simulink model "XplaneControlInterface"  (R2024b)
settings: Solver=FixedStepAuto  StartTime=0.0  StopTime=inf  FixedStep=0.02  RelTol=1e-3
libraries: dspnetwork x3, instrumentseriallib x2, etargetslib x2, sldrtlib x2, svdutilitieslib x1, slpidlib x1
settings Model: PacingRate=10  Creator=정예린  LastModifiedBy=banana99ou
settings RTWCC: GPUComputeCapability=3.5

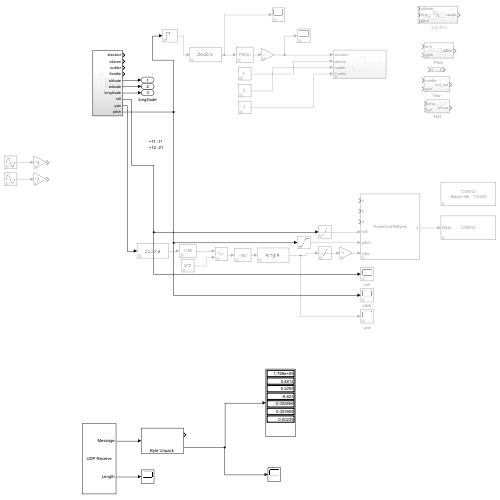
[thumbnail: Simulink's stored preview of the top-level diagram]
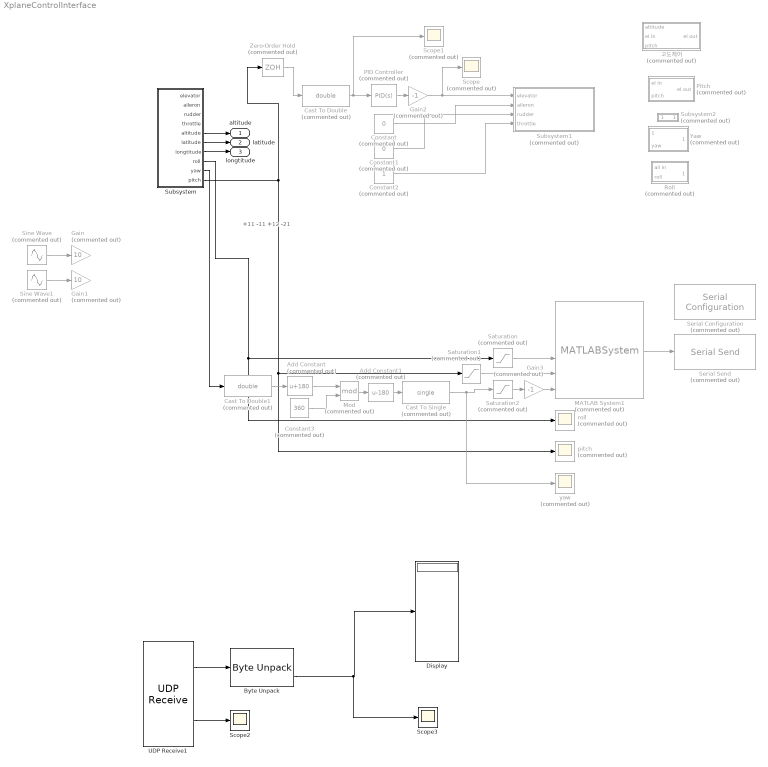
== system XplaneControlInterface ==
  note: +11 -11
      | +12 -21
  Add Constant : Bias  Commented=on  Bias=180  SaturateOnIntegerOverflow=off
  Add Constant1 : Bias  Commented=on  Bias=-180  SaturateOnIntegerOverflow=off
  Byte Unpack : svdutilitieslib/Byte Unpack  dimensions={[1],[7]}  datatypes={'single','single'}  byteAlign=4  blockPlatform=arduinoert
  Cast To Double : DataTypeConversion  Commented=on  OutDataTypeStr=double  SaturateOnIntegerOverflow=off  RndMeth=Floor
  Cast To Double1 : DataTypeConversion  Commented=on  OutDataTypeStr=double  SaturateOnIntegerOverflow=off  RndMeth=Floor
  Cast To Single : DataTypeConversion  Commented=on  OutDataTypeStr=single  SaturateOnIntegerOverflow=off  RndMeth=Floor
  Constant : Constant  Commented=on  Value=0
  Constant1 : Constant  Commented=on  Value=0
  Constant2 : Constant  Commented=on
  Constant3 : Constant  Commented=on  Value=360
  Display : Display
  Gain : Gain  Commented=on  Gain=10
  Gain1 : Gain  Commented=on  Gain=10
  Gain2 : Gain  Commented=on  Gain=-1
  Gain3 : Gain  Commented=on  Gain=-1
  MATLAB System1 : MATLABSystem  Commented=on  System=PoseCmdToBytes  Precision=3  MaxLen=128  PadByte=10  SimulateUsing=Code generation
      mask Type: PoseCmdToBytes
      mask Display:
      | disp('PoseCmdToBytes');
      | port_label('input',1,'x');
      | port_label('input',2,'y');
      | port_label('input',3,'z');
      | port_label('input',4,'roll');
      | port_label('input',5,'pitch');
      | port_label('input',6,'yaw');
      | port_label('output',1,'y');
  Mod : Math  Commented=on  Operator=mod
  PID Controller : slpidlib/PID Controller  Commented=on  Controller=PID  Form=Parallel  TimeDomain=Continuous-time  UseExternalTs=off  SampleTime=-1  IntegratorMethod=Forward Euler  FilterMethod=Forward Euler  ControllerParametersSource=internal  P=4  I=0  UseKiTs=off  D=0  UseExternalDerivativeSource=off  N=100  UseFilter=on  TunerSelectOption=Transfer Function Based (PID Tuner App)  InitialConditionSource=internal  InitialConditionForIntegrator=0  InitialConditionForFilter=0  DifferentiatorICPrevScaledInput=0  ExternalReset=none  TrackingMode=off  Kt=1  LimitOutput=off  SatLimitsSource=internal  UpperSaturationLimit=inf  LowerSaturationLimit=-inf  LinearizeAsGain=on  AntiWindupMode=none  Kb=1  LimitIntegrator=off  UpperIntegratorSaturationLimit=inf  LowerIntegratorSaturationLimit=-inf  POutMin=[]  POutMax=[]  IOutMin=[]  IOutMax=[]  DOutMin=[]  DOutMax=[]  NOutMin=[]  NOutMax=[]  SumOutMin=[]  SumOutMax=[]  SaturationOutMin=[]  SaturationOutMax=[]  PParamMin=[]  PParamMax=[]  IParamMin=[]  IParamMax=[]  DParamMin=[]  DParamMax=[]  NParamMin=[]  NParamMax=[]  KbParamMin=[]  KbParamMax=[]  KtParamMin=[]  KtParamMax=[]  KbOutMin=[]  KbOutMax=[]  KtOutMin=[]  KtOutMax=[]  IntegratorOutMin=[]  IntegratorOutMax=[]  FilterOutMin=[]  FilterOutMax=[]  SumI1OutMin=[]  SumI1OutMax=[]  SumI2OutMin=[]  SumI2OutMax=[]  SumI3OutMin=[]  SumI3OutMax=[]  SumI4OutMin=[]  SumI4OutMax=[]  SumDOutMin=[]  SumDOutMax=[]  DifferentiatorOutMin=[]  DifferentiatorOutMax=[]  FilterDiffOutCoefMin=[]  FilterDiffOutCoefMax=[]  ReciprocalOutMin=[]  ReciprocalOutMax=[]  SumDenOutMin=[]  SumDenOutMax=[]  SumNumOutMin=[]  SumNumOutMax=[]  DivideOutMin=[]  DivideOutMax=[]  UdiffTsProdOutMin=[]  UdiffTsProdOutMax=[]  NTsProdOutMin=[]  NTsProdOutMax=[]  UintegralTsProdOutMin=[]  UintegralTsProdOutMax=[]  UngainTsProdOutMin=[]  UngainTsProdOutMax=[]  ClampingZeroOutDataTypeStr=Inherit: Inherit via back propagation  ClampingZeroOutMin=[]  ClampingZeroOutMax=[]  FilterDenConstantOutDataTypeStr=Inherit: Inherit via back propagation  FilterDenConstantOutMin=[]  FilterDenConstantOutMax=[]  PCopyOutDataTypeStr=Inherit: Inherit via back propagation  PCopyOutMin=[]  PCopyOutMax=[]  NCopyOutDataTypeStr=Inherit: Inherit via back propagation  NCopyOutMin=[]  NCopyOutMax=[]  IntegratorContinuousStateAttributes=''  IntegratorStateMustResolveToSignalObject=off  IntegratorRTWStateStorageClass=Auto  FilterContinuousStateAttributes=''  FilterStateMustResolveToSignalObject=off  FilterRTWStateStorageClass=Auto  ParallelPVariant=InternalParameters  IdealPVariant=Disabled  IVariant=InternalParameters  DVariant=InternalParameters  IntegratorVariant=Continuous  SatVariant=Disabled  AWVariant=Passthrough  PCopyVariant=Disabled  TRVariant=Disabled  FdbkBlocksVariant=Forward  IdealPFdbkVariant=Disabled  SatFdbkVariant=Disabled  DerivativeFilterVariant=ContFilter  NVariant=InternalParameters  NCopyVariant=Disabled  FilterICVariant=InternalICsFilter  IntegratorICVariant=InternalICs  ExternalResetVariant=Disabled  TRSumVariant=Passthrough  SumFdbkVariant=Disabled  SumVariant=Sum_PID  TsampFilterVariant=InternalTs  TsampNgainVariant=Passthrough  TsampIntegralVariant=Disabled_SignalSpec  ExternalSaturationOutDataTypeStr=Inherit: Same as second input  DerivativeSourceVariant=ErrorSignal  PreIntVariant=InternalPreInt
  Pitch : Subsystem  Commented=on
  Roll : Subsystem  Commented=on
  Saturation : Saturate  Commented=on  UpperLimit=11  LowerLimit=-11
  Saturation1 : Saturate  Commented=on  UpperLimit=12  LowerLimit=-21
  Saturation2 : Saturate  Commented=on  UpperLimit=20  LowerLimit=-20
  Scope : Scope  Commented=on
  Scope1 : Scope  Commented=on
  Scope2 : Scope
  Scope3 : Scope
  Serial Configuration : instrumentseriallib/Serial Configuration  Priority=-200000  Commented=on  PortSel=COM12  Port=COM12  ComPort=COM12  BaudRate=115200  DataBits=8  Parity=none  StopBits=1  ByteOrder=little-endian  FlowControl=none  Timeout=10  SimulateUsing=Interpreted execution  BlockInModel=on  aMode=1
  Serial Send : instrumentseriallib/Serial Send  Priority=1  Commented=on  PortSel=COM12  Port=COM12  ComPort=COM12  Header=[]  Terminator=<none>  CustomTerminator=[]  EnableBlockingMode=on  SimulateUsing=Interpreted execution  BlockInModel=on  aMode=1
  Sine Wave : Sin  Commented=on  Frequency=0.25  SampleTime=0
  Sine Wave1 : Sin  Commented=on  Frequency=0.25  Phase=1.5708  SampleTime=0
  Subsystem : Subsystem
  Subsystem1 : Subsystem  Commented=on
  Subsystem2 : Subsystem  Commented=on
  UDP Receive1 : dspnetwork/UDP Receive  localURL='0.0.0.0'  localPort=32901  remoteURL='0.0.0.0'  remotePort=-1  recvBufferSize=8192  dims=32  signalDatatype=uint8  isComplex=off  isVarSize=off  showBlockingTime=off  blockingTime=0  sampletime=inf  blockPlatform=[]
  Yaw : Subsystem  Commented=on
  Zero-Order Hold : ZeroOrderHold  Commented=on  SampleTime=-1
  pitch : Scope  Commented=on
  roll : Scope  Commented=on
  yaw : Scope  Commented=on
  고도제어 : Subsystem  Commented=on
  altitude : Outport
  latitude : Outport  Port=2
  longtitude : Outport  Port=3
  wires:
  MATLAB System1/1 -> Serial Send/1
  Sine Wave/1 -> Gain/1
  Sine Wave1/1 -> Gain1/1
  Subsystem/8(roll) -> roll/1, Saturation/1
  Subsystem/10(pitch) -> Zero-Order Hold/1, pitch/1, Saturation1/1
  Subsystem/7(longtitude) -> longtitude/1
  Subsystem/6(latitude) -> latitude/1
  Subsystem/5(altitude) -> altitude/1
  Constant/1 -> Subsystem1/2(aileron)
  Constant1/1 -> Subsystem1/3(rudder)
  Constant2/1 -> Subsystem1/4(throttle)
  PID Controller/1 -> Gain2/1
  Cast To Double/1 -> Scope1/1, PID Controller/1
  Zero-Order Hold/1 -> Cast To Double/1
  Gain2/1 -> Scope/1, Subsystem1/1(elevator)
  Saturation/1 -> MATLAB System1/4
  Saturation2/1 -> Gain3/1
  Saturation1/1 -> MATLAB System1/5
  Subsystem/9(yaw) -> Cast To Double1/1
  Mod/1 -> Add Constant1/1
  Add Constant/1 -> Mod/1
  Constant3/1 -> Mod/2
  Cast To Double1/1 -> Add Constant/1
  Cast To Single/1 -> yaw/1, Saturation2/1
  Add Constant1/1 -> Cast To Single/1
  Gain3/1 -> MATLAB System1/6
  UDP Receive1/1 -> Byte Unpack/1
  UDP Receive1/2 -> Scope2/1
  Byte Unpack/2 -> Scope3/1, Display/1

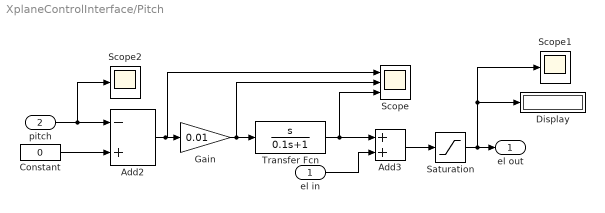
== system XplaneControlInterface/Pitch ==
  el in : Inport
  pitch : Inport  Port=2
  Add2 : Sum  Inputs=-+
  Add3 : Sum
  Constant : Constant  Value=0
  Display : Display
  Gain : Gain  Gain=0.01
  Saturation : Saturate  UpperLimit=1  LowerLimit=-1
  Scope : Scope  NumInputPorts=3
  Scope1 : Scope
  Scope2 : Scope
  Transfer Fcn : TransferFcn  Numerator=[1 0]  Denominator=[0.1 1]
  el out : Outport
  wires:
  el in/1 -> Add3/2
  Add3/1 -> Saturation/1
  Saturation/1 -> Scope1/1, Display/1, el out/1
  Gain/1 -> Scope/2, Transfer Fcn/1
  Add2/1 -> Scope/1, Gain/1
  Transfer Fcn/1 -> Scope/3, Add3/1
  Constant/1 -> Add2/2
  pitch/1 -> Scope2/1, Add2/1

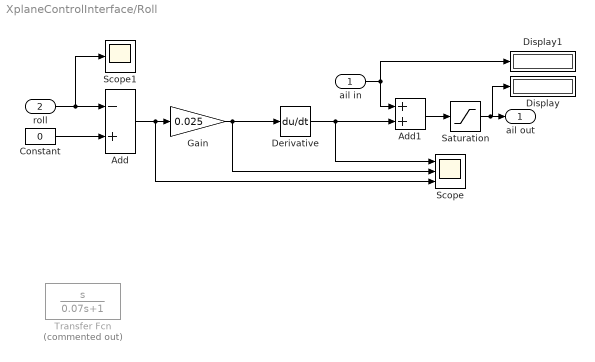
== system XplaneControlInterface/Roll ==
  ail in : Inport
  roll : Inport  Port=2
  Add : Sum  Inputs=-+
  Add1 : Sum
  Constant : Constant  Value=0
  Derivative : Derivative  CoefficientInTFapproximation=0.07
  Display : Display
  Display1 : Display
  Gain : Gain  Gain=0.025
  Saturation : Saturate  UpperLimit=1  LowerLimit=-1
  Scope : Scope  NumInputPorts=3
  Scope1 : Scope
  Transfer Fcn : TransferFcn  Commented=on  Numerator=[1 0]  Denominator=[0.07 1]
  ail out : Outport
  wires:
  Constant/1 -> Add/2
  Add/1 -> Scope/3, Gain/1
  Add1/1 -> Saturation/1
  ail in/1 -> Add1/1, Display1/1
  Saturation/1 -> ail out/1, Display/1
  roll/1 -> Scope1/1, Add/1
  Gain/1 -> Derivative/1, Scope/2
  Derivative/1 -> Scope/1, Add1/2

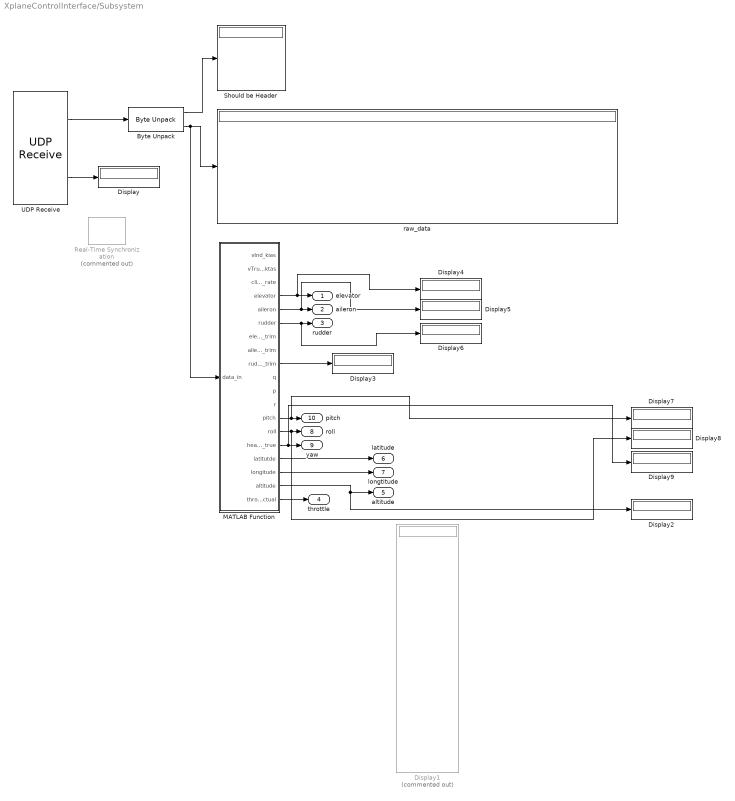
== system XplaneControlInterface/Subsystem ==
  Byte Unpack : etargetslib/Byte Unpack  dimensions={5,[9,8]}  datatypes={'uint8','single'}  byteAlign=1
  Display{,2..9} (9 alike) : Display
  Display1 : Display  Commented=on
  MATLAB Function : MATLAB Function  TreatAsAtomicUnit=on
  Real-Time Synchronization : sldrtlib/Real-Time Synchronization  Commented=on  SampleTime=0.1  MaxMissedTicks=10  ShowMissedTicks=off  YieldWhenWaiting=off
  Should be Header : Display
  UDP Receive : dspnetwork/UDP Receive  localURL='0.0.0.0'  localPort=49004  remoteURL='127.0.0.1'  remotePort=-1  recvBufferSize=8192  dims=293  signalDatatype=uint8  isComplex=off  isVarSize=off  showBlockingTime=off  blockingTime=0  sampletime=inf  blockPlatform=[]
  raw_data : Display
  elevator : Outport
  aileron : Outport  Port=2
  rudder : Outport  Port=3
  throttle : Outport  Port=4
  altitude : Outport  Port=5
  latitude : Outport  Port=6
  longtitude : Outport  Port=7
  roll : Outport  Port=8
  yaw : Outport  Port=9
  pitch : Outport  Port=10
  wires:
  Byte Unpack/1 -> Should be Header/1
  Byte Unpack/2 -> MATLAB Function/1(data_in), raw_data/1
  UDP Receive/2 -> Display/1
  UDP Receive/1 -> Byte Unpack/1
  MATLAB Function/4(elevator) -> Display4/1, elevator/1
  MATLAB Function/5(aileron) -> Display5/1, aileron/1
  MATLAB Function/6(rudder) -> Display6/1, rudder/1
  MATLAB Function/18(altitude) -> altitude/1, Display2/1
  MATLAB Function/19(throttle_actual) -> throttle/1
  MATLAB Function/16(latitutde) -> latitude/1
  MATLAB Function/17(longitude) -> longtitude/1
  MATLAB Function/14(roll) -> Display8/1, roll/1
  MATLAB Function/15(heading_true) -> Display9/1, yaw/1
  MATLAB Function/9(rudder_trim) -> Display3/1
  MATLAB Function/13(pitch) -> Display7/1, pitch/1

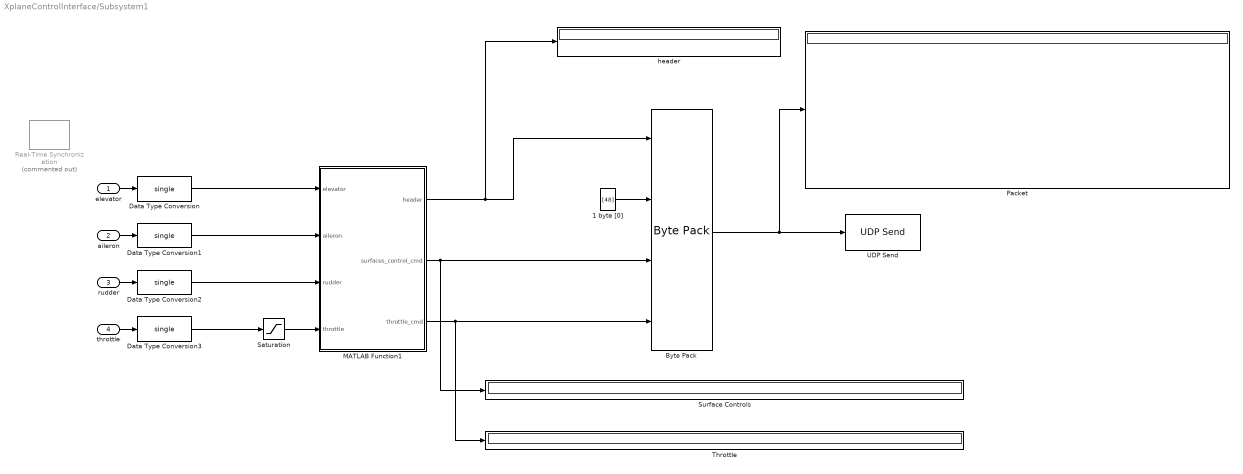
== system XplaneControlInterface/Subsystem1 ==
  elevator : Inport
  aileron : Inport  Port=2
  rudder : Inport  Port=3
  throttle : Inport  Port=4
  1 byte [0] : Constant  Value=[48]  OutDataTypeStr=uint8
  Byte Pack : etargetslib/Byte Pack  datatypes={'uint8','uint8','single','single'}  byteAlign=1
  Data Type Conversion{,1..3} (4 alike) : DataTypeConversion  OutDataTypeStr=single  SaturateOnIntegerOverflow=off  RndMeth=Floor
  MATLAB Function1 : MATLAB Function  TreatAsAtomicUnit=on
  Packet : Display
  Real-Time Synchronization : sldrtlib/Real-Time Synchronization  Commented=on  SampleTime=0.1  MaxMissedTicks=10  ShowMissedTicks=off  YieldWhenWaiting=off
  Saturation : Saturate  UpperLimit=1  LowerLimit=0
  Surface Controls : Display
  Throttle : Display
  UDP Send : dspnetwork/UDP Send  remoteURL='127.0.0.1'  remotePort=49000  localURL='0.0.0.0'  localPortSource=Automatically determine  localPort=-1  sendBufferSize=8192  sampletime=-1  blockPlatform=[]  separateLengthPort=0
  header : Display
  wires:
  MATLAB Function1/2(surfaces_control_cmd) -> Surface Controls/1, Byte Pack/3
  Saturation/1 -> MATLAB Function1/4(throttle)
  MATLAB Function1/1(header) -> Byte Pack/1, header/1
  1 byte [0]/1 -> Byte Pack/2
  Byte Pack/1 -> UDP Send/1, Packet/1
  MATLAB Function1/3(throttle_cmd) -> Throttle/1, Byte Pack/4
  elevator/1 -> Data Type Conversion/1
  aileron/1 -> Data Type Conversion1/1
  Data Type Conversion1/1 -> MATLAB Function1/2(aileron)
  rudder/1 -> Data Type Conversion2/1
  Data Type Conversion2/1 -> MATLAB Function1/3(rudder)
  throttle/1 -> Data Type Conversion3/1
  Data Type Conversion3/1 -> Saturation/1
  Data Type Conversion/1 -> MATLAB Function1/1(elevator)

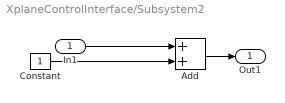
== system XplaneControlInterface/Subsystem2 ==
  In1 : Inport
  Add : Sum
  Constant : Constant
  Out1 : Outport
  wires:
  Constant/1 -> Add/2
  Add/1 -> Out1/1
  In1/1 -> Add/1

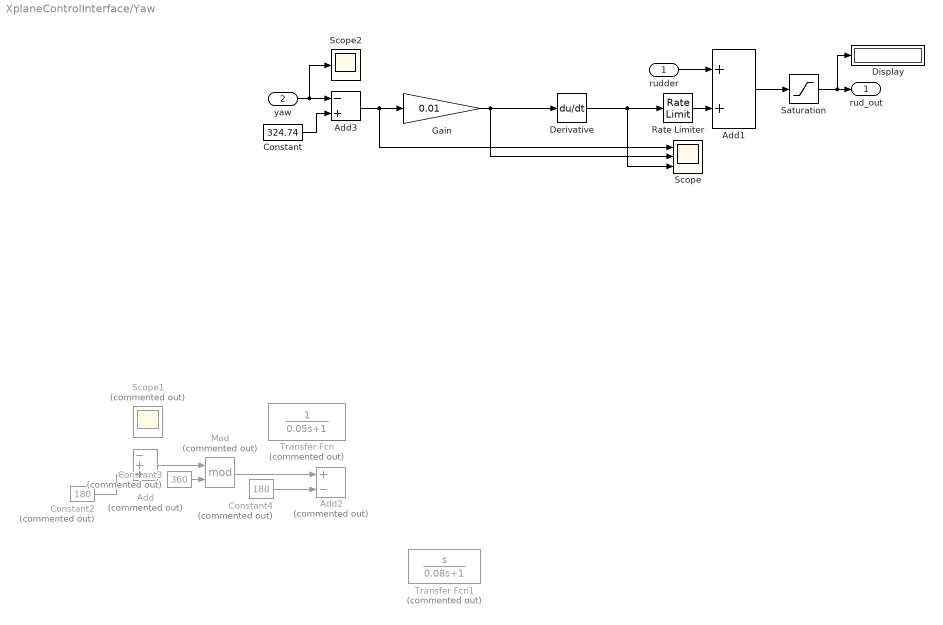
== system XplaneControlInterface/Yaw ==
  rudder : Inport
  yaw : Inport  Port=2
  Add : Sum  Commented=on  Inputs=-++
  Add1 : Sum
  Add2 : Sum  Commented=on  Inputs=+-
  Add3 : Sum  Inputs=-+
  Constant : Constant  Value=324.74
  Constant2 : Constant  Commented=on  Value=180
  Constant3 : Constant  Commented=on  Value=360
  Constant4 : Constant  Commented=on  Value=180
  Derivative : Derivative  CoefficientInTFapproximation=0.08
  Display : Display
  Gain : Gain  Gain=0.01
  Mod : Math  Commented=on  Operator=mod
  Rate Limiter : RateLimiter  RisingSlewLimit=0.5  FallingSlewLimit=-0.5  SampleTimeMode=inherited
  Saturation : Saturate  UpperLimit=1  LowerLimit=-1
  Scope : Scope  NumInputPorts=3
  Scope1 : Scope  Commented=on
  Scope2 : Scope
  Transfer Fcn : TransferFcn  Commented=on  Denominator=[0.05 1]
  Transfer Fcn1 : TransferFcn  Commented=on  Numerator=[1 0]  Denominator=[0.08 1]
  rud_out : Outport
  wires:
  Add1/1 -> Saturation/1
  rudder/1 -> Add1/1
  Saturation/1 -> Display/1, rud_out/1
  Gain/1 -> Derivative/1, Scope/2
  Constant2/1 -> Add/3
  Add/1 -> Mod/1
  Constant3/1 -> Mod/2
  Mod/1 -> Add2/1
  Constant4/1 -> Add2/2
  Add3/1 -> Scope/1, Gain/1
  yaw/1 -> Scope2/1, Add3/1
  Constant/1 -> Add3/2
  Rate Limiter/1 -> Add1/2
  Derivative/1 -> Scope/3, Rate Limiter/1

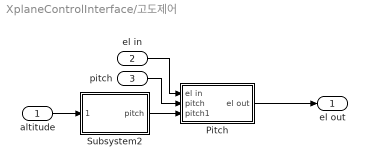
== system XplaneControlInterface/고도제어 ==
  altitude : Inport
  el in : Inport  Port=2
  pitch : Inport  Port=3
  Pitch : Subsystem
  Subsystem2 : Subsystem
  el out : Outport
  wires:
  Pitch/1(el out) -> el out/1
  Subsystem2/1(" pitch") -> Pitch/3(pitch1)
  altitude/1 -> Subsystem2/1(altitude)
  el in/1 -> Pitch/1(el in)
  pitch/1 -> Pitch/2(pitch)

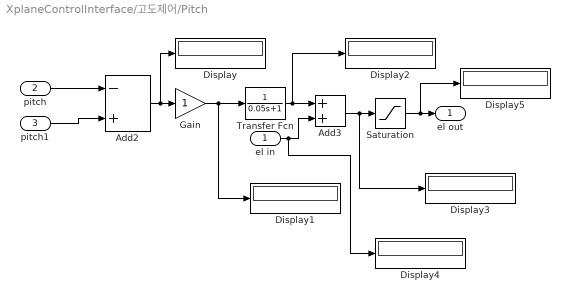
== system XplaneControlInterface/고도제어/Pitch ==
  el in : Inport
  pitch : Inport  Port=2
  pitch1 : Inport  Port=3
  Add2 : Sum  Inputs=-+
  Add3 : Sum
  Display{,1..5} (6 alike) : Display
  Gain : Gain
  Saturation : Saturate  UpperLimit=1  LowerLimit=-1
  Transfer Fcn : TransferFcn  Denominator=[0.05 1]
  el out : Outport
  wires:
  el in/1 -> Display4/1, Add3/2
  Add3/1 -> Display3/1, Saturation/1
  pitch1/1 -> Add2/2
  Saturation/1 -> Display5/1, el out/1
  Gain/1 -> Transfer Fcn/1, Display1/1
  Add2/1 -> Display/1, Gain/1
  Transfer Fcn/1 -> Display2/1, Add3/1
  pitch/1 -> Add2/1

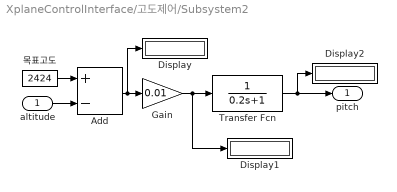
== system XplaneControlInterface/고도제어/Subsystem2 ==
  altitude : Inport
  Add : Sum  Inputs=+-
  Display : Display
  Display1 : Display
  Display2 : Display
  Gain : Gain  Gain=0.01
  Transfer Fcn : TransferFcn  Denominator=[0.2 1]
  목표고도 : Constant  Value=2424
  " pitch" : Outport
  wires:
  목표고도/1 -> Add/1
  altitude/1 -> Add/2
  Add/1 -> Display/1, Gain/1
  Gain/1 -> Transfer Fcn/1, Display1/1
  Transfer Fcn/1 -> Display2/1, " pitch"/1

== matlab function XplaneControlInterface/Subsystem1/MATLAB Function1 ==
  data: elevator input; header output uint8; surfaces_control_cmd output; aileron input single; rudder input single; throttle input; throttle_cmd output single
function [header,surfaces_control_cmd,throttle_cmd] = fcn(elevator, aileron, rudder, throttle) 
header =[uint8(68) uint8(65) uint8(84) uint8(65)];
No_Comand = single(-999);
 %Surface_header = typecast(uint8([uint8(8) uint8(0) uint8(0) uint8(0)]),'single')
surfaces_control_cmd = [1.1210388e-44 elevator aileron rudder No_Comand No_Comand No_Comand No_Comand No_Comand  ];
%Throttle_header = typecast(uint8([uint8(25) uint8(0) uint8(0) uint8(0)]),'single');
throttle_cmd = [3.503246160812043e-44 throttle No_Comand No_Comand No_Comand No_Comand No_Comand No_Comand No_Comand];
end

== matlab function XplaneControlInterface/Subsystem/MATLAB Function ==
  data: data_in input; vInd_kias output; vTrue_ktas output; climb_rate output; elevator output; aileron output; rudder output; elevator_trim output; aileron_trim output; rudder_trim output; q output; p output; r output; pitch output; roll output; heading_true output; latitutde output; longitude output; altitude output; throttle_actual output
function [vInd_kias,vTrue_ktas,...
    climb_rate,...
    elevator,aileron,rudder,...
    elevator_trim,aileron_trim,rudder_trim,...
    q,p,r,...
    pitch, roll, heading_true,...
    latitutde, longitude, altitude,...
    throttle_actual] = decoder(data_in)
 vInd_kias = data_in(2,1);
 vTrue_ktas = data_in(4,1);
 climb_rate = data_in(4,2);
 elevator = data_in(2,4);
 aileron = data_in(3,4);
 rudder= data_in(4,4);
 elevator_trim= data_in(2,7);
 aileron_trim= data_in(3,7);
 rudder_trim= data_in(4,7);
 q= data_in(2,5);
 p= data_in(3,5);
 r= data_in(4,5);
 pitch= data_in(2,2);
 roll= data_in(3,2);
 heading_true= data_in(4,2);
 latitutde= data_in(2,4);
 longitude= data_in(3,4);
 altitude= data_in(7,4);
 throttle_actual = data_in(2,6);
end
